simulink model "Lab1_4B"  (R2018a)
settings: Solver=VariableStepAuto  StartTime=0.0  StopTime=30  RelTol=1e-9
settings Model: Creator=melab2  LastModifiedBy=melab2

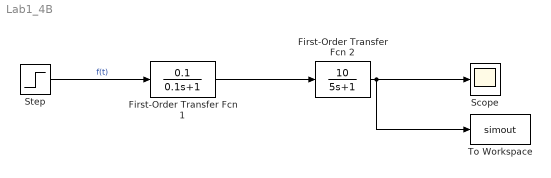
== system Lab1_4B ==
  First-Order Transfer Fcn 1 : TransferFcn  Numerator=[0.1]  Denominator=[0.1 1]
  First-Order Transfer Fcn 2 : TransferFcn  Numerator=[10]  Denominator=[5 1]
  "Scope " : Scope
  "Step " : Step  SampleTime=0
  "To Workspace " : ToWorkspace  VariableName=simout  SampleTime=-1
  wires:
  "Step "/1 -> First-Order Transfer Fcn 1/1  "f(t)"
  First-Order Transfer Fcn 1/1 -> First-Order Transfer Fcn 2/1
  First-Order Transfer Fcn 2/1 -> "To Workspace "/1, "Scope "/1
